simulink model "PitchAttitudeHold_ModernControlS"  (R2024b)
settings: Solver=VariableStepAuto  StartTime=0.0  StopTime=25  RelTol=1e-3
values from neighbouring files (symbols this model uses):
  K = lqr(A,B,Q,R)    [PitchAttitudeHold_ModernControl.m]    (also in RollAngleHold_ModernControl.m = place(A, B, eigs))
  sysKf = ss(A - Kf*C, [B Kf], eye(4), 0*[B Kf])    [PitchAttitudeHold_ModernControl.m]
  sysLong = ss(A,B,C,D,'statename',states,'inputname',inputs,'outputname',outputs)    [AltitudeHold_ModernControl.m]    (also in PitchAttitudeHold_ModernControl.m = ss(A,B,C,D))
settings Model: Creator=wangdi  LastModifiedBy=wangdi

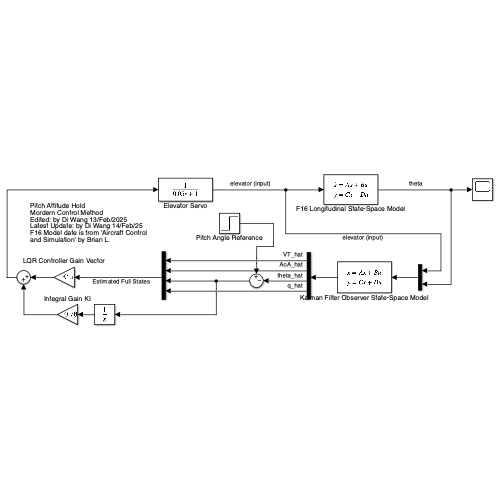
[thumbnail: Simulink's stored preview of the top-level diagram]
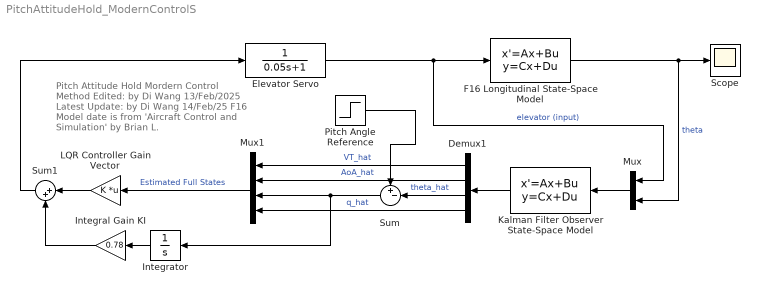
== system PitchAttitudeHold_ModernControlS ==
  note: Pitch Attitude Hold
      | Mordern Control Method
      | Edited: by Di Wang 13/Feb/2025
      | Latest Update: by Di Wang 14/Feb/25
      | F16 Model date is from 'Aircraft Control and Simulation' by Brian L.
  Demux1 : Demux
  Elevator Servo : TransferFcn  Denominator=[0.05 1]
  F16 Longitudinal State-Space Model : StateSpace  A=sysLong.A  B=sysLong.B  C=sysLong.C  D=sysLong.D  InitialCondition=0
  Integral Gain KI : Gain  Gain=0.78
  Integrator : Integrator
  Kalman Filter Observer State-Space Model : StateSpace  A=sysKf.A  B=sysKf.B  C=sysKf.C  D=sysKf.D  InitialCondition=0
  LQR Controller Gain Vector : Gain  Gain=K  Multiplication=Matrix(K*u)
  Mux : Mux  Inputs=2
  Mux1 : Mux
  Pitch Angle Reference : Step  SampleTime=0
  Scope : Scope
  Sum : Sum  Inputs=+-|
  Sum1 : Sum  Inputs=|++
  wires:
  Mux/1 -> Kalman Filter Observer State-Space Model/1
  Kalman Filter Observer State-Space Model/1 -> Demux1/1
  Demux1/4 -> Mux1/4  "q_hat"
  Demux1/2 -> Mux1/2  "AoA_hat"
  Demux1/1 -> Mux1/1  "VT_hat"
  Mux1/1 -> LQR Controller Gain Vector/1  "Estimated Full States"
  Pitch Angle Reference/1 -> Sum/1
  Sum/1 -> Integrator/1, Mux1/3
  Demux1/3 -> Sum/2  "theta_hat"
  Elevator Servo/1 -> Mux/1, F16 Longitudinal State-Space Model/1  "elevator (input)"
  Sum1/1 -> Elevator Servo/1
  F16 Longitudinal State-Space Model/1 -> Mux/2, Scope/1  "theta"
  Integrator/1 -> Integral Gain KI/1
  LQR Controller Gain Vector/1 -> Sum1/1
  Integral Gain KI/1 -> Sum1/2
